simulink model "Gen_net_5"  (R2018b)
settings: Solver=FixedStepAuto  StartTime=0.0  StopTime=100  FixedStep=0.1  RelTol=1e-3
undefined symbols (not defined in the file): g, Jx, Jy, Jz, m, phi_DoS_duration_1, phi_DoS_duration_2, phi_DoS_duration_3, phi_DoS_duration_4, phi_DoS_duration_5, phi_FDI_value_1, phi_FDI_value_2, phi_FDI_value_3, phi_FDI_value_4, phi_FDI_value_5, phi_Replay_delay_1, phi_Replay_delay_2, phi_Replay_delay_3, phi_Replay_delay_4, phi_Replay_delay_5, psi_DoS_duration_1, psi_DoS_duration_2, psi_DoS_duration_3, psi_DoS_duration_4, psi_DoS_duration_5, psi_FDI_value_1, psi_FDI_value_2, psi_FDI_value_3, psi_FDI_value_4, psi_FDI_value_5, psi_Replay_delay_1, psi_Replay_delay_2, psi_Replay_delay_3, psi_Replay_delay_4, psi_Replay_delay_5, T_DoS_duration_1, T_DoS_duration_2, T_DoS_duration_3, T_DoS_duration_4, T_DoS_duration_5, T_FDI_value_1, T_FDI_value_2, T_FDI_value_3, T_FDI_value_4, T_FDI_value_5, T_Replay_delay_1, T_Replay_delay_2, T_Replay_delay_3, T_Replay_delay_4, T_Replay_delay_5, tau_phi_DoS_duration_1, tau_phi_DoS_duration_2, tau_phi_DoS_duration_3, tau_phi_DoS_duration_4, tau_phi_DoS_duration_5, tau_phi_FDI_value_1, tau_phi_FDI_value_2, tau_phi_FDI_value_3, tau_phi_FDI_value_4, tau_phi_FDI_value_5 ... (+95)
libraries: simulink x30
(part 3 of 4)

== system Gen_net_5/quad 2/quadcopter/S(7-9) ==
  phi : Inport
  theta : Inport  Port=2
  q : Inport  Port=3
  P : Inport  Port=4
  r : Inport  Port=5
  Add2 : Sum  Inputs=++-
  Add3 : Sum
  Cos{6..9} (4 alike) : Trigonometry  Operator=cos
  Multiply3 : Product  Inputs=3
  Multiply4 : Product  Inputs=3
  Multiply5 : Product  Inputs=**/
  Multiply6 : Product  Inputs=**/
  Product5 : Product
  Product6 : Product
  Sin6 : Trigonometry
  Sin7 : Trigonometry
  Sin8 : Trigonometry
  Sin9 : Trigonometry  Operator=cos
  Subtract1 : Sum  Inputs=-+
  Tan : Trigonometry  Operator=tan
  Tan1 : Trigonometry  Operator=tan
  Out1 : Outport
  Out2 : Outport  Port=2
  Out3 : Outport  Port=3
  wires:
  Multiply5/1 -> Subtract1/1
  q/1 -> Multiply5/1, Product5/1, Multiply4/3
  phi/1 -> Sin9/1, Sin8/1, Sin7/1, Cos7/1, Cos6/1, Sin6/1
  Multiply4/1 -> Add2/2
  theta/1 -> Cos9/1, Cos8/1, Tan/1, Tan1/1
  Tan/1 -> Multiply4/2
  r/1 -> Multiply6/1, Product6/1, Multiply3/3
  Multiply6/1 -> Subtract1/2
  Sin9/1 -> Multiply6/2
  Sin6/1 -> Multiply4/1
  Sin8/1 -> Multiply5/2
  Tan1/1 -> Multiply3/2
  Product5/1 -> Add3/1
  Cos6/1 -> Multiply3/1
  Product6/1 -> Add3/2
  Sin7/1 -> Product6/2
  Multiply3/1 -> Add2/3
  Cos7/1 -> Product5/2
  Cos8/1 -> Multiply5/3
  Cos9/1 -> Multiply6/3
  Subtract1/1 -> Out3/1
  P/1 -> Add2/1
  Add2/1 -> Out1/1
  Add3/1 -> Out2/1

== system Gen_net_5/quad 3/controller/altitude controller ==
  z_ref : Inport
  z : Inport  Port=2
  Constant : Constant  Value=m*g
  PID Controller : simulink/Continuous/PID Controller  Controller=PID  Form=Parallel  TimeDomain=Continuous-time  SampleTime=-1  IntegratorMethod=Forward Euler  FilterMethod=Forward Euler  ControllerParametersSource=internal  P=0.995151437850186  I=0.128436617904908  D=1.76652121748459  UseFilter=on  N=3.43027649580308  TunerSelectOption=Transfer Function Based (PID Tuner App)  InitialConditionSource=internal  InitialConditionForIntegrator=0  InitialConditionForFilter=0  DifferentiatorICPrevScaledInput=0  ExternalReset=none  TrackingMode=off  Kt=1  LimitOutput=off  UpperSaturationLimit=inf  LowerSaturationLimit=-inf  LinearizeAsGain=on  AntiWindupMode=none  Kb=1  POutMin=[]  POutMax=[]  IOutMin=[]  IOutMax=[]  DOutMin=[]  DOutMax=[]  NOutMin=[]  NOutMax=[]  SumOutMin=[]  SumOutMax=[]  SaturationOutMin=[]  SaturationOutMax=[]  PParamMin=[]  PParamMax=[]  IParamMin=[]  IParamMax=[]  DParamMin=[]  DParamMax=[]  NParamMin=[]  NParamMax=[]  KbParamMin=[]  KbParamMax=[]  KtParamMin=[]  KtParamMax=[]  KbOutMin=[]  KbOutMax=[]  KtOutMin=[]  KtOutMax=[]  IntegratorOutMin=[]  IntegratorOutMax=[]  FilterOutMin=[]  FilterOutMax=[]  SumI1OutMin=[]  SumI1OutMax=[]  SumI2OutMin=[]  SumI2OutMax=[]  SumI3OutMin=[]  SumI3OutMax=[]  SumI4OutMin=[]  SumI4OutMax=[]  SumDOutMin=[]  SumDOutMax=[]  DifferentiatorOutMin=[]  DifferentiatorOutMax=[]  FilterDiffOutCoefMin=[]  FilterDiffOutCoefMax=[]  ReciprocalOutMin=[]  ReciprocalOutMax=[]  SumDenOutMin=[]  SumDenOutMax=[]  SumNumOutMin=[]  SumNumOutMax=[]  DivideOutMin=[]  DivideOutMax=[]  IntegratorContinuousStateAttributes=''  IntegratorStateMustResolveToSignalObject=off  IntegratorRTWStateStorageClass=Auto  FilterContinuousStateAttributes=''  FilterStateMustResolveToSignalObject=off  FilterRTWStateStorageClass=Auto  ParallelPVariant=InternalParameters  IdealPVariant=Disabled  IVariant=InternalParameters  DVariant=InternalParameters  IntegratorVariant=Continuous  SatVariant=Disabled  AWVariant=Passthrough  PCopyVariant=Disabled  TRVariant=Disabled  FdbkBlocksVariant=Forward  IdealPFdbkVariant=Disabled  SatFdbkVariant=Disabled  DerivativeFilterVariant=ContFilter  NVariant=InternalParameters  NCopyVariant=Disabled  FilterICVariant=InternalICsFilter  IntegratorICVariant=InternalICs  ExternalResetVariant=Disabled  TRSumVariant=Passthrough  SumFdbkVariant=Disabled  SumVariant=Sum_PID
  Sum1 : Sum  Inputs=++|
  Sum2 : Sum  Inputs=-+|
  T : Outport
  wires:
  z_ref/1 -> Sum2/2  "z_ref"
  Sum2/1 -> PID Controller/1  "z_err"
  z/1 -> Sum2/1  "z"
  PID Controller/1 -> Sum1/2
  Sum1/1 -> T/1  "z_err"
  Constant/1 -> Sum1/1

== system Gen_net_5/quad 3/controller/attitude controller ==
  phi : Inport
  theta : Inport  Port=2
  phi_ref : Inport  Port=3
  theta_ref : Inport  Port=4
  PID Controller1 : simulink/Continuous/PID Controller  Controller=PID  Form=Parallel  TimeDomain=Continuous-time  SampleTime=-1  IntegratorMethod=Forward Euler  FilterMethod=Forward Euler  ControllerParametersSource=internal  P=0.00283727985172173  I=0.000300746607233676  D=0.00592713753900793  UseFilter=on  N=3.27588862149554  TunerSelectOption=Transfer Function Based (PID Tuner App)  InitialConditionSource=internal  InitialConditionForIntegrator=0  InitialConditionForFilter=0  DifferentiatorICPrevScaledInput=0  ExternalReset=none  TrackingMode=off  Kt=1  LimitOutput=off  UpperSaturationLimit=inf  LowerSaturationLimit=-inf  LinearizeAsGain=on  AntiWindupMode=none  Kb=1  POutMin=[]  POutMax=[]  IOutMin=[]  IOutMax=[]  DOutMin=[]  DOutMax=[]  NOutMin=[]  NOutMax=[]  SumOutMin=[]  SumOutMax=[]  SaturationOutMin=[]  SaturationOutMax=[]  PParamMin=[]  PParamMax=[]  IParamMin=[]  IParamMax=[]  DParamMin=[]  DParamMax=[]  NParamMin=[]  NParamMax=[]  KbParamMin=[]  KbParamMax=[]  KtParamMin=[]  KtParamMax=[]  KbOutMin=[]  KbOutMax=[]  KtOutMin=[]  KtOutMax=[]  IntegratorOutMin=[]  IntegratorOutMax=[]  FilterOutMin=[]  FilterOutMax=[]  SumI1OutMin=[]  SumI1OutMax=[]  SumI2OutMin=[]  SumI2OutMax=[]  SumI3OutMin=[]  SumI3OutMax=[]  SumI4OutMin=[]  SumI4OutMax=[]  SumDOutMin=[]  SumDOutMax=[]  DifferentiatorOutMin=[]  DifferentiatorOutMax=[]  FilterDiffOutCoefMin=[]  FilterDiffOutCoefMax=[]  ReciprocalOutMin=[]  ReciprocalOutMax=[]  SumDenOutMin=[]  SumDenOutMax=[]  SumNumOutMin=[]  SumNumOutMax=[]  DivideOutMin=[]  DivideOutMax=[]  IntegratorContinuousStateAttributes=''  IntegratorStateMustResolveToSignalObject=off  IntegratorRTWStateStorageClass=Auto  FilterContinuousStateAttributes=''  FilterStateMustResolveToSignalObject=off  FilterRTWStateStorageClass=Auto  ParallelPVariant=InternalParameters  IdealPVariant=Disabled  IVariant=InternalParameters  DVariant=InternalParameters  IntegratorVariant=Continuous  SatVariant=Disabled  AWVariant=Passthrough  PCopyVariant=Disabled  TRVariant=Disabled  FdbkBlocksVariant=Forward  IdealPFdbkVariant=Disabled  SatFdbkVariant=Disabled  DerivativeFilterVariant=ContFilter  NVariant=InternalParameters  NCopyVariant=Disabled  FilterICVariant=InternalICsFilter  IntegratorICVariant=InternalICs  ExternalResetVariant=Disabled  TRSumVariant=Passthrough  SumFdbkVariant=Disabled  SumVariant=Sum_PID
  PID Controller2 : simulink/Continuous/PID Controller  Controller=PID  Form=Parallel  TimeDomain=Continuous-time  SampleTime=-1  IntegratorMethod=Forward Euler  FilterMethod=Forward Euler  ControllerParametersSource=internal  P=0.00376352907272366  I=0.000541941810599823  D=0.00599672187002239  UseFilter=on  N=3.43027649580308  TunerSelectOption=Transfer Function Based (PID Tuner App)  InitialConditionSource=internal  InitialConditionForIntegrator=0  InitialConditionForFilter=0  DifferentiatorICPrevScaledInput=0  ExternalReset=none  TrackingMode=off  Kt=1  LimitOutput=off  UpperSaturationLimit=inf  LowerSaturationLimit=-inf  LinearizeAsGain=on  AntiWindupMode=none  Kb=1  POutMin=[]  POutMax=[]  IOutMin=[]  IOutMax=[]  DOutMin=[]  DOutMax=[]  NOutMin=[]  NOutMax=[]  SumOutMin=[]  SumOutMax=[]  SaturationOutMin=[]  SaturationOutMax=[]  PParamMin=[]  PParamMax=[]  IParamMin=[]  IParamMax=[]  DParamMin=[]  DParamMax=[]  NParamMin=[]  NParamMax=[]  KbParamMin=[]  KbParamMax=[]  KtParamMin=[]  KtParamMax=[]  KbOutMin=[]  KbOutMax=[]  KtOutMin=[]  KtOutMax=[]  IntegratorOutMin=[]  IntegratorOutMax=[]  FilterOutMin=[]  FilterOutMax=[]  SumI1OutMin=[]  SumI1OutMax=[]  SumI2OutMin=[]  SumI2OutMax=[]  SumI3OutMin=[]  SumI3OutMax=[]  SumI4OutMin=[]  SumI4OutMax=[]  SumDOutMin=[]  SumDOutMax=[]  DifferentiatorOutMin=[]  DifferentiatorOutMax=[]  FilterDiffOutCoefMin=[]  FilterDiffOutCoefMax=[]  ReciprocalOutMin=[]  ReciprocalOutMax=[]  SumDenOutMin=[]  SumDenOutMax=[]  SumNumOutMin=[]  SumNumOutMax=[]  DivideOutMin=[]  DivideOutMax=[]  IntegratorContinuousStateAttributes=''  IntegratorStateMustResolveToSignalObject=off  IntegratorRTWStateStorageClass=Auto  FilterContinuousStateAttributes=''  FilterStateMustResolveToSignalObject=off  FilterRTWStateStorageClass=Auto  ParallelPVariant=InternalParameters  IdealPVariant=Disabled  IVariant=InternalParameters  DVariant=InternalParameters  IntegratorVariant=Continuous  SatVariant=Disabled  AWVariant=Passthrough  PCopyVariant=Disabled  TRVariant=Disabled  FdbkBlocksVariant=Forward  IdealPFdbkVariant=Disabled  SatFdbkVariant=Disabled  DerivativeFilterVariant=ContFilter  NVariant=InternalParameters  NCopyVariant=Disabled  FilterICVariant=InternalICsFilter  IntegratorICVariant=InternalICs  ExternalResetVariant=Disabled  TRSumVariant=Passthrough  SumFdbkVariant=Disabled  SumVariant=Sum_PID
  Sum1 : Sum  Inputs=-+|
  Sum2 : Sum  Inputs=-+|
  tau_phi : Outport
  tau_theta : Outport  Port=2
  wires:
  phi/1 -> Sum2/1
  theta/1 -> Sum1/1
  phi_ref/1 -> Sum2/2
  theta_ref/1 -> Sum1/2
  Sum1/1 -> PID Controller2/1
  PID Controller2/1 -> tau_theta/1
  Sum2/1 -> PID Controller1/1
  PID Controller1/1 -> tau_phi/1

== system Gen_net_5/quad 3/controller/position controller ==
  x_ref : Inport
  x : Inport  Port=2
  y_ref : Inport  Port=3
  y : Inport  Port=4
  PID Controller : simulink/Continuous/PID Controller  Controller=PID  Form=Parallel  TimeDomain=Continuous-time  SampleTime=-1  IntegratorMethod=Forward Euler  FilterMethod=Forward Euler  ControllerParametersSource=internal  P=-0.0353666022144165  I=-0.000286794158433156  D=-0.0628063352706131  UseFilter=on  N=2.54551622754876  TunerSelectOption=Transfer Function Based (PID Tuner App)  InitialConditionSource=internal  InitialConditionForIntegrator=0  InitialConditionForFilter=0  DifferentiatorICPrevScaledInput=0  ExternalReset=none  TrackingMode=off  Kt=1  LimitOutput=off  UpperSaturationLimit=inf  LowerSaturationLimit=-inf  LinearizeAsGain=on  AntiWindupMode=none  Kb=1  POutMin=[]  POutMax=[]  IOutMin=[]  IOutMax=[]  DOutMin=[]  DOutMax=[]  NOutMin=[]  NOutMax=[]  SumOutMin=[]  SumOutMax=[]  SaturationOutMin=[]  SaturationOutMax=[]  PParamMin=[]  PParamMax=[]  IParamMin=[]  IParamMax=[]  DParamMin=[]  DParamMax=[]  NParamMin=[]  NParamMax=[]  KbParamMin=[]  KbParamMax=[]  KtParamMin=[]  KtParamMax=[]  KbOutMin=[]  KbOutMax=[]  KtOutMin=[]  KtOutMax=[]  IntegratorOutMin=[]  IntegratorOutMax=[]  FilterOutMin=[]  FilterOutMax=[]  SumI1OutMin=[]  SumI1OutMax=[]  SumI2OutMin=[]  SumI2OutMax=[]  SumI3OutMin=[]  SumI3OutMax=[]  SumI4OutMin=[]  SumI4OutMax=[]  SumDOutMin=[]  SumDOutMax=[]  DifferentiatorOutMin=[]  DifferentiatorOutMax=[]  FilterDiffOutCoefMin=[]  FilterDiffOutCoefMax=[]  ReciprocalOutMin=[]  ReciprocalOutMax=[]  SumDenOutMin=[]  SumDenOutMax=[]  SumNumOutMin=[]  SumNumOutMax=[]  DivideOutMin=[]  DivideOutMax=[]  IntegratorContinuousStateAttributes=''  IntegratorStateMustResolveToSignalObject=off  IntegratorRTWStateStorageClass=Auto  FilterContinuousStateAttributes=''  FilterStateMustResolveToSignalObject=off  FilterRTWStateStorageClass=Auto  ParallelPVariant=InternalParameters  IdealPVariant=Disabled  IVariant=InternalParameters  DVariant=InternalParameters  IntegratorVariant=Continuous  SatVariant=Disabled  AWVariant=Passthrough  PCopyVariant=Disabled  TRVariant=Disabled  FdbkBlocksVariant=Forward  IdealPFdbkVariant=Disabled  SatFdbkVariant=Disabled  DerivativeFilterVariant=ContFilter  NVariant=InternalParameters  NCopyVariant=Disabled  FilterICVariant=InternalICsFilter  IntegratorICVariant=InternalICs  ExternalResetVariant=Disabled  TRSumVariant=Passthrough  SumFdbkVariant=Disabled  SumVariant=Sum_PID
  PID Controller1 : simulink/Continuous/PID Controller  Controller=PID  Form=Parallel  TimeDomain=Continuous-time  SampleTime=-1  IntegratorMethod=Forward Euler  FilterMethod=Forward Euler  ControllerParametersSource=internal  P=0.0344011339376346  I=0.00030706355489176  D=0.0770084502146799  UseFilter=on  N=2.81850869669594  TunerSelectOption=Transfer Function Based (PID Tuner App)  InitialConditionSource=internal  InitialConditionForIntegrator=0  InitialConditionForFilter=0  DifferentiatorICPrevScaledInput=0  ExternalReset=none  TrackingMode=off  Kt=1  LimitOutput=off  UpperSaturationLimit=inf  LowerSaturationLimit=-inf  LinearizeAsGain=on  AntiWindupMode=none  Kb=1  POutMin=[]  POutMax=[]  IOutMin=[]  IOutMax=[]  DOutMin=[]  DOutMax=[]  NOutMin=[]  NOutMax=[]  SumOutMin=[]  SumOutMax=[]  SaturationOutMin=[]  SaturationOutMax=[]  PParamMin=[]  PParamMax=[]  IParamMin=[]  IParamMax=[]  DParamMin=[]  DParamMax=[]  NParamMin=[]  NParamMax=[]  KbParamMin=[]  KbParamMax=[]  KtParamMin=[]  KtParamMax=[]  KbOutMin=[]  KbOutMax=[]  KtOutMin=[]  KtOutMax=[]  IntegratorOutMin=[]  IntegratorOutMax=[]  FilterOutMin=[]  FilterOutMax=[]  SumI1OutMin=[]  SumI1OutMax=[]  SumI2OutMin=[]  SumI2OutMax=[]  SumI3OutMin=[]  SumI3OutMax=[]  SumI4OutMin=[]  SumI4OutMax=[]  SumDOutMin=[]  SumDOutMax=[]  DifferentiatorOutMin=[]  DifferentiatorOutMax=[]  FilterDiffOutCoefMin=[]  FilterDiffOutCoefMax=[]  ReciprocalOutMin=[]  ReciprocalOutMax=[]  SumDenOutMin=[]  SumDenOutMax=[]  SumNumOutMin=[]  SumNumOutMax=[]  DivideOutMin=[]  DivideOutMax=[]  IntegratorContinuousStateAttributes=''  IntegratorStateMustResolveToSignalObject=off  IntegratorRTWStateStorageClass=Auto  FilterContinuousStateAttributes=''  FilterStateMustResolveToSignalObject=off  FilterRTWStateStorageClass=Auto  ParallelPVariant=InternalParameters  IdealPVariant=Disabled  IVariant=InternalParameters  DVariant=InternalParameters  IntegratorVariant=Continuous  SatVariant=Disabled  AWVariant=Passthrough  PCopyVariant=Disabled  TRVariant=Disabled  FdbkBlocksVariant=Forward  IdealPFdbkVariant=Disabled  SatFdbkVariant=Disabled  DerivativeFilterVariant=ContFilter  NVariant=InternalParameters  NCopyVariant=Disabled  FilterICVariant=InternalICsFilter  IntegratorICVariant=InternalICs  ExternalResetVariant=Disabled  TRSumVariant=Passthrough  SumFdbkVariant=Disabled  SumVariant=Sum_PID
  Sum1 : Sum  Inputs=-+|
  Sum2 : Sum  Inputs=-+|
  phi_ref : Outport
  theta_ref : Outport  Port=2
  wires:
  x_ref/1 -> Sum2/2
  x/1 -> Sum2/1
  Sum2/1 -> PID Controller/1
  PID Controller/1 -> theta_ref/1
  Sum1/1 -> PID Controller1/1
  y_ref/1 -> Sum1/2
  y/1 -> Sum1/1
  PID Controller1/1 -> phi_ref/1

== system Gen_net_5/quad 3/controller/yaw controller ==
  yaw : Inport
  Constant : Constant  Value=0
  PID Controller3 : simulink/Continuous/PID Controller  Controller=PID  Form=Parallel  TimeDomain=Continuous-time  SampleTime=-1  IntegratorMethod=Forward Euler  FilterMethod=Forward Euler  ControllerParametersSource=internal  P=0.00651371850229212  I=0.000840676044468491  D=0.0115626843326264  UseFilter=on  N=3.43027649580308  TunerSelectOption=Transfer Function Based (PID Tuner App)  InitialConditionSource=internal  InitialConditionForIntegrator=0  InitialConditionForFilter=0  DifferentiatorICPrevScaledInput=0  ExternalReset=none  TrackingMode=off  Kt=1  LimitOutput=off  UpperSaturationLimit=inf  LowerSaturationLimit=-inf  LinearizeAsGain=on  AntiWindupMode=none  Kb=1  POutMin=[]  POutMax=[]  IOutMin=[]  IOutMax=[]  DOutMin=[]  DOutMax=[]  NOutMin=[]  NOutMax=[]  SumOutMin=[]  SumOutMax=[]  SaturationOutMin=[]  SaturationOutMax=[]  PParamMin=[]  PParamMax=[]  IParamMin=[]  IParamMax=[]  DParamMin=[]  DParamMax=[]  NParamMin=[]  NParamMax=[]  KbParamMin=[]  KbParamMax=[]  KtParamMin=[]  KtParamMax=[]  KbOutMin=[]  KbOutMax=[]  KtOutMin=[]  KtOutMax=[]  IntegratorOutMin=[]  IntegratorOutMax=[]  FilterOutMin=[]  FilterOutMax=[]  SumI1OutMin=[]  SumI1OutMax=[]  SumI2OutMin=[]  SumI2OutMax=[]  SumI3OutMin=[]  SumI3OutMax=[]  SumI4OutMin=[]  SumI4OutMax=[]  SumDOutMin=[]  SumDOutMax=[]  DifferentiatorOutMin=[]  DifferentiatorOutMax=[]  FilterDiffOutCoefMin=[]  FilterDiffOutCoefMax=[]  ReciprocalOutMin=[]  ReciprocalOutMax=[]  SumDenOutMin=[]  SumDenOutMax=[]  SumNumOutMin=[]  SumNumOutMax=[]  DivideOutMin=[]  DivideOutMax=[]  IntegratorContinuousStateAttributes=''  IntegratorStateMustResolveToSignalObject=off  IntegratorRTWStateStorageClass=Auto  FilterContinuousStateAttributes=''  FilterStateMustResolveToSignalObject=off  FilterRTWStateStorageClass=Auto  ParallelPVariant=InternalParameters  IdealPVariant=Disabled  IVariant=InternalParameters  DVariant=InternalParameters  IntegratorVariant=Continuous  SatVariant=Disabled  AWVariant=Passthrough  PCopyVariant=Disabled  TRVariant=Disabled  FdbkBlocksVariant=Forward  IdealPFdbkVariant=Disabled  SatFdbkVariant=Disabled  DerivativeFilterVariant=ContFilter  NVariant=InternalParameters  NCopyVariant=Disabled  FilterICVariant=InternalICsFilter  IntegratorICVariant=InternalICs  ExternalResetVariant=Disabled  TRSumVariant=Passthrough  SumFdbkVariant=Disabled  SumVariant=Sum_PID
  Sum2 : Sum  Inputs=-+|
  tau_psi : Outport
  wires:
  yaw/1 -> Sum2/1
  Constant/1 -> Sum2/2
  Sum2/1 -> PID Controller3/1
  PID Controller3/1 -> tau_psi/1

== system Gen_net_5/quad 3/quadcopter/S(10-12) ==
  q : Inport
  P : Inport  Port=2
  r : Inport  Port=3
  In4 : Inport  Port=4
  In5 : Inport  Port=5
  In6 : Inport  Port=6
  Add4 : Sum
  Add5 : Sum
  Add6 : Sum
  Constant4 : Constant  Value=(Jy - Jz) / Jx
  Constant5 : Constant  Value=Jx
  Constant6 : Constant  Value=(Jz - Jx) / Jy
  Constant7 : Constant  Value=Jy
  Constant8 : Constant  Value=(Jx - Jy) / Jz
  Constant9 : Constant  Value=Jz
  Multiply10 : Product  Inputs=*/
  Multiply11 : Product  Inputs=*/
  Multiply12 : Product  Inputs=3
  Multiply7 : Product  Inputs=3
  Multiply8 : Product  Inputs=*/
  Multiply9 : Product  Inputs=3
  Out1 : Outport
  Out2 : Outport  Port=2
  Out3 : Outport  Port=3
  wires:
  r/1 -> Multiply9/3, Multiply7/3
  Constant8/1 -> Multiply12/1
  In5/1 -> Multiply10/1
  Multiply8/1 -> Add4/2
  Multiply7/1 -> Add4/1
  Constant7/1 -> Multiply10/2
  Constant5/1 -> Multiply8/2
  Constant4/1 -> Multiply7/1
  q/1 -> Multiply7/2, Multiply12/3
  Multiply10/1 -> Add5/2
  Multiply9/1 -> Add5/1
  Constant9/1 -> Multiply11/2
  In6/1 -> Multiply11/1
  Constant6/1 -> Multiply9/1
  Multiply12/1 -> Add6/1
  P/1 -> Multiply9/2, Multiply12/2
  In4/1 -> Multiply8/1
  Multiply11/1 -> Add6/2
  Add4/1 -> Out1/1
  Add5/1 -> Out2/1
  Add6/1 -> Out3/1

== system Gen_net_5/quad 3/quadcopter/S(4-6) ==
  In1 : Inport
  phi : Inport  Port=2
  theta : Inport  Port=3
  psi : Inport  Port=4
  Add : Sum  Inputs=--
  Add1 : Sum  Inputs=+-
  Constant1 : Constant  Value=0.0
  Constant3 : Constant  Value=g
  Cos{,1..5} (6 alike) : Trigonometry  Operator=cos
  Multiply : Product
  Multiply1 : Product
  Multiply2 : Product
  Product : Product  Inputs=3
  Product1 : Product
  Product2 : Product
  Product3 : Product  Inputs=3
  Product4 : Product
  Sin{,1..5} (6 alike) : Trigonometry
  Subtract : Sum  Inputs=+-
  Sum3 : Sum  Inputs=++|
  Out1 : Outport
  Out2 : Outport  Port=2
  Out3 : Outport  Port=3
  wires:
  phi/1 -> Cos4/1, Cos3/1, Cos1/1, Sin2/1, Sin3/1
  theta/1 -> Sin/1, Sin5/1, Cos5/1
  Sum3/1 -> Out1/1
  Constant1/1 -> Sum3/1
  Product1/1 -> Add/2
  Sin3/1 -> Product2/2
  Cos/1 -> Product/1
  Cos1/1 -> Product/3
  Multiply/1 -> Sum3/2
  Sin/1 -> Product/2
  Cos5/1 -> Product4/2
  psi/1 -> Cos/1, Sin1/1, Cos2/1, Sin4/1
  Cos3/1 -> Product3/3
  Product2/1 -> Add1/1
  Add1/1 -> Multiply1/2
  Sin1/1 -> Product1/1
  Sin4/1 -> Product3/1
  Sin5/1 -> Product3/2
  Cos4/1 -> Product4/1
  Cos2/1 -> Product2/1
  Subtract/1 -> Out3/1
  Sin2/1 -> Product1/2
  Constant3/1 -> Subtract/2
  Product4/1 -> Multiply2/2
  In1/1 -> Multiply2/1, Multiply1/1, Multiply/1
  Add/1 -> Multiply/2
  Product3/1 -> Add1/2
  Multiply2/1 -> Subtract/1
  Product/1 -> Add/1
  Multiply1/1 -> Out2/1

== system Gen_net_5/quad 3/quadcopter/S(7-9) ==
  phi : Inport
  theta : Inport  Port=2
  q : Inport  Port=3
  P : Inport  Port=4
  r : Inport  Port=5
  Add2 : Sum  Inputs=++-
  Add3 : Sum
  Cos{6..9} (4 alike) : Trigonometry  Operator=cos
  Multiply3 : Product  Inputs=3
  Multiply4 : Product  Inputs=3
  Multiply5 : Product  Inputs=**/
  Multiply6 : Product  Inputs=**/
  Product5 : Product
  Product6 : Product
  Sin6 : Trigonometry
  Sin7 : Trigonometry
  Sin8 : Trigonometry
  Sin9 : Trigonometry  Operator=cos
  Subtract1 : Sum  Inputs=-+
  Tan : Trigonometry  Operator=tan
  Tan1 : Trigonometry  Operator=tan
  Out1 : Outport
  Out2 : Outport  Port=2
  Out3 : Outport  Port=3
  wires:
  Multiply5/1 -> Subtract1/1
  q/1 -> Multiply5/1, Product5/1, Multiply4/3
  phi/1 -> Sin9/1, Sin8/1, Sin7/1, Cos7/1, Cos6/1, Sin6/1
  Multiply4/1 -> Add2/2
  theta/1 -> Cos9/1, Cos8/1, Tan/1, Tan1/1
  Tan/1 -> Multiply4/2
  r/1 -> Multiply6/1, Product6/1, Multiply3/3
  Multiply6/1 -> Subtract1/2
  Sin9/1 -> Multiply6/2
  Sin6/1 -> Multiply4/1
  Sin8/1 -> Multiply5/2
  Tan1/1 -> Multiply3/2
  Product5/1 -> Add3/1
  Cos6/1 -> Multiply3/1
  Product6/1 -> Add3/2
  Sin7/1 -> Product6/2
  Multiply3/1 -> Add2/3
  Cos7/1 -> Product5/2
  Cos8/1 -> Multiply5/3
  Cos9/1 -> Multiply6/3
  Subtract1/1 -> Out3/1
  P/1 -> Add2/1
  Add2/1 -> Out1/1
  Add3/1 -> Out2/1

== system Gen_net_5/quad 4/controller/altitude controller ==
  z_ref : Inport
  z : Inport  Port=2
  Constant : Constant  Value=m*g
  PID Controller : simulink/Continuous/PID Controller  Controller=PID  Form=Parallel  TimeDomain=Continuous-time  SampleTime=-1  IntegratorMethod=Forward Euler  FilterMethod=Forward Euler  ControllerParametersSource=internal  P=0.995151437850186  I=0.128436617904908  D=1.76652121748459  UseFilter=on  N=3.43027649580308  TunerSelectOption=Transfer Function Based (PID Tuner App)  InitialConditionSource=internal  InitialConditionForIntegrator=0  InitialConditionForFilter=0  DifferentiatorICPrevScaledInput=0  ExternalReset=none  TrackingMode=off  Kt=1  LimitOutput=off  UpperSaturationLimit=inf  LowerSaturationLimit=-inf  LinearizeAsGain=on  AntiWindupMode=none  Kb=1  POutMin=[]  POutMax=[]  IOutMin=[]  IOutMax=[]  DOutMin=[]  DOutMax=[]  NOutMin=[]  NOutMax=[]  SumOutMin=[]  SumOutMax=[]  SaturationOutMin=[]  SaturationOutMax=[]  PParamMin=[]  PParamMax=[]  IParamMin=[]  IParamMax=[]  DParamMin=[]  DParamMax=[]  NParamMin=[]  NParamMax=[]  KbParamMin=[]  KbParamMax=[]  KtParamMin=[]  KtParamMax=[]  KbOutMin=[]  KbOutMax=[]  KtOutMin=[]  KtOutMax=[]  IntegratorOutMin=[]  IntegratorOutMax=[]  FilterOutMin=[]  FilterOutMax=[]  SumI1OutMin=[]  SumI1OutMax=[]  SumI2OutMin=[]  SumI2OutMax=[]  SumI3OutMin=[]  SumI3OutMax=[]  SumI4OutMin=[]  SumI4OutMax=[]  SumDOutMin=[]  SumDOutMax=[]  DifferentiatorOutMin=[]  DifferentiatorOutMax=[]  FilterDiffOutCoefMin=[]  FilterDiffOutCoefMax=[]  ReciprocalOutMin=[]  ReciprocalOutMax=[]  SumDenOutMin=[]  SumDenOutMax=[]  SumNumOutMin=[]  SumNumOutMax=[]  DivideOutMin=[]  DivideOutMax=[]  IntegratorContinuousStateAttributes=''  IntegratorStateMustResolveToSignalObject=off  IntegratorRTWStateStorageClass=Auto  FilterContinuousStateAttributes=''  FilterStateMustResolveToSignalObject=off  FilterRTWStateStorageClass=Auto  ParallelPVariant=InternalParameters  IdealPVariant=Disabled  IVariant=InternalParameters  DVariant=InternalParameters  IntegratorVariant=Continuous  SatVariant=Disabled  AWVariant=Passthrough  PCopyVariant=Disabled  TRVariant=Disabled  FdbkBlocksVariant=Forward  IdealPFdbkVariant=Disabled  SatFdbkVariant=Disabled  DerivativeFilterVariant=ContFilter  NVariant=InternalParameters  NCopyVariant=Disabled  FilterICVariant=InternalICsFilter  IntegratorICVariant=InternalICs  ExternalResetVariant=Disabled  TRSumVariant=Passthrough  SumFdbkVariant=Disabled  SumVariant=Sum_PID
  Sum1 : Sum  Inputs=++|
  Sum2 : Sum  Inputs=-+|
  T : Outport
  wires:
  z_ref/1 -> Sum2/2  "z_ref"
  Sum2/1 -> PID Controller/1  "z_err"
  z/1 -> Sum2/1  "z"
  PID Controller/1 -> Sum1/2
  Sum1/1 -> T/1  "z_err"
  Constant/1 -> Sum1/1

== system Gen_net_5/quad 4/controller/attitude controller ==
  phi : Inport
  theta : Inport  Port=2
  phi_ref : Inport  Port=3
  theta_ref : Inport  Port=4
  PID Controller1 : simulink/Continuous/PID Controller  Controller=PID  Form=Parallel  TimeDomain=Continuous-time  SampleTime=-1  IntegratorMethod=Forward Euler  FilterMethod=Forward Euler  ControllerParametersSource=internal  P=0.00283727985172173  I=0.000300746607233676  D=0.00592713753900793  UseFilter=on  N=3.27588862149554  TunerSelectOption=Transfer Function Based (PID Tuner App)  InitialConditionSource=internal  InitialConditionForIntegrator=0  InitialConditionForFilter=0  DifferentiatorICPrevScaledInput=0  ExternalReset=none  TrackingMode=off  Kt=1  LimitOutput=off  UpperSaturationLimit=inf  LowerSaturationLimit=-inf  LinearizeAsGain=on  AntiWindupMode=none  Kb=1  POutMin=[]  POutMax=[]  IOutMin=[]  IOutMax=[]  DOutMin=[]  DOutMax=[]  NOutMin=[]  NOutMax=[]  SumOutMin=[]  SumOutMax=[]  SaturationOutMin=[]  SaturationOutMax=[]  PParamMin=[]  PParamMax=[]  IParamMin=[]  IParamMax=[]  DParamMin=[]  DParamMax=[]  NParamMin=[]  NParamMax=[]  KbParamMin=[]  KbParamMax=[]  KtParamMin=[]  KtParamMax=[]  KbOutMin=[]  KbOutMax=[]  KtOutMin=[]  KtOutMax=[]  IntegratorOutMin=[]  IntegratorOutMax=[]  FilterOutMin=[]  FilterOutMax=[]  SumI1OutMin=[]  SumI1OutMax=[]  SumI2OutMin=[]  SumI2OutMax=[]  SumI3OutMin=[]  SumI3OutMax=[]  SumI4OutMin=[]  SumI4OutMax=[]  SumDOutMin=[]  SumDOutMax=[]  DifferentiatorOutMin=[]  DifferentiatorOutMax=[]  FilterDiffOutCoefMin=[]  FilterDiffOutCoefMax=[]  ReciprocalOutMin=[]  ReciprocalOutMax=[]  SumDenOutMin=[]  SumDenOutMax=[]  SumNumOutMin=[]  SumNumOutMax=[]  DivideOutMin=[]  DivideOutMax=[]  IntegratorContinuousStateAttributes=''  IntegratorStateMustResolveToSignalObject=off  IntegratorRTWStateStorageClass=Auto  FilterContinuousStateAttributes=''  FilterStateMustResolveToSignalObject=off  FilterRTWStateStorageClass=Auto  ParallelPVariant=InternalParameters  IdealPVariant=Disabled  IVariant=InternalParameters  DVariant=InternalParameters  IntegratorVariant=Continuous  SatVariant=Disabled  AWVariant=Passthrough  PCopyVariant=Disabled  TRVariant=Disabled  FdbkBlocksVariant=Forward  IdealPFdbkVariant=Disabled  SatFdbkVariant=Disabled  DerivativeFilterVariant=ContFilter  NVariant=InternalParameters  NCopyVariant=Disabled  FilterICVariant=InternalICsFilter  IntegratorICVariant=InternalICs  ExternalResetVariant=Disabled  TRSumVariant=Passthrough  SumFdbkVariant=Disabled  SumVariant=Sum_PID
  PID Controller2 : simulink/Continuous/PID Controller  Controller=PID  Form=Parallel  TimeDomain=Continuous-time  SampleTime=-1  IntegratorMethod=Forward Euler  FilterMethod=Forward Euler  ControllerParametersSource=internal  P=0.00376352907272366  I=0.000541941810599823  D=0.00599672187002239  UseFilter=on  N=3.43027649580308  TunerSelectOption=Transfer Function Based (PID Tuner App)  InitialConditionSource=internal  InitialConditionForIntegrator=0  InitialConditionForFilter=0  DifferentiatorICPrevScaledInput=0  ExternalReset=none  TrackingMode=off  Kt=1  LimitOutput=off  UpperSaturationLimit=inf  LowerSaturationLimit=-inf  LinearizeAsGain=on  AntiWindupMode=none  Kb=1  POutMin=[]  POutMax=[]  IOutMin=[]  IOutMax=[]  DOutMin=[]  DOutMax=[]  NOutMin=[]  NOutMax=[]  SumOutMin=[]  SumOutMax=[]  SaturationOutMin=[]  SaturationOutMax=[]  PParamMin=[]  PParamMax=[]  IParamMin=[]  IParamMax=[]  DParamMin=[]  DParamMax=[]  NParamMin=[]  NParamMax=[]  KbParamMin=[]  KbParamMax=[]  KtParamMin=[]  KtParamMax=[]  KbOutMin=[]  KbOutMax=[]  KtOutMin=[]  KtOutMax=[]  IntegratorOutMin=[]  IntegratorOutMax=[]  FilterOutMin=[]  FilterOutMax=[]  SumI1OutMin=[]  SumI1OutMax=[]  SumI2OutMin=[]  SumI2OutMax=[]  SumI3OutMin=[]  SumI3OutMax=[]  SumI4OutMin=[]  SumI4OutMax=[]  SumDOutMin=[]  SumDOutMax=[]  DifferentiatorOutMin=[]  DifferentiatorOutMax=[]  FilterDiffOutCoefMin=[]  FilterDiffOutCoefMax=[]  ReciprocalOutMin=[]  ReciprocalOutMax=[]  SumDenOutMin=[]  SumDenOutMax=[]  SumNumOutMin=[]  SumNumOutMax=[]  DivideOutMin=[]  DivideOutMax=[]  IntegratorContinuousStateAttributes=''  IntegratorStateMustResolveToSignalObject=off  IntegratorRTWStateStorageClass=Auto  FilterContinuousStateAttributes=''  FilterStateMustResolveToSignalObject=off  FilterRTWStateStorageClass=Auto  ParallelPVariant=InternalParameters  IdealPVariant=Disabled  IVariant=InternalParameters  DVariant=InternalParameters  IntegratorVariant=Continuous  SatVariant=Disabled  AWVariant=Passthrough  PCopyVariant=Disabled  TRVariant=Disabled  FdbkBlocksVariant=Forward  IdealPFdbkVariant=Disabled  SatFdbkVariant=Disabled  DerivativeFilterVariant=ContFilter  NVariant=InternalParameters  NCopyVariant=Disabled  FilterICVariant=InternalICsFilter  IntegratorICVariant=InternalICs  ExternalResetVariant=Disabled  TRSumVariant=Passthrough  SumFdbkVariant=Disabled  SumVariant=Sum_PID
  Sum1 : Sum  Inputs=-+|
  Sum2 : Sum  Inputs=-+|
  tau_phi : Outport
  tau_theta : Outport  Port=2
  wires:
  phi/1 -> Sum2/1
  theta/1 -> Sum1/1
  phi_ref/1 -> Sum2/2
  theta_ref/1 -> Sum1/2
  Sum1/1 -> PID Controller2/1
  PID Controller2/1 -> tau_theta/1
  Sum2/1 -> PID Controller1/1
  PID Controller1/1 -> tau_phi/1

== system Gen_net_5/quad 4/controller/position controller ==
  x_ref : Inport
  x : Inport  Port=2
  y_ref : Inport  Port=3
  y : Inport  Port=4
  PID Controller : simulink/Continuous/PID Controller  Controller=PID  Form=Parallel  TimeDomain=Continuous-time  SampleTime=-1  IntegratorMethod=Forward Euler  FilterMethod=Forward Euler  ControllerParametersSource=internal  P=-0.0353666022144165  I=-0.000286794158433156  D=-0.0628063352706131  UseFilter=on  N=2.54551622754876  TunerSelectOption=Transfer Function Based (PID Tuner App)  InitialConditionSource=internal  InitialConditionForIntegrator=0  InitialConditionForFilter=0  DifferentiatorICPrevScaledInput=0  ExternalReset=none  TrackingMode=off  Kt=1  LimitOutput=off  UpperSaturationLimit=inf  LowerSaturationLimit=-inf  LinearizeAsGain=on  AntiWindupMode=none  Kb=1  POutMin=[]  POutMax=[]  IOutMin=[]  IOutMax=[]  DOutMin=[]  DOutMax=[]  NOutMin=[]  NOutMax=[]  SumOutMin=[]  SumOutMax=[]  SaturationOutMin=[]  SaturationOutMax=[]  PParamMin=[]  PParamMax=[]  IParamMin=[]  IParamMax=[]  DParamMin=[]  DParamMax=[]  NParamMin=[]  NParamMax=[]  KbParamMin=[]  KbParamMax=[]  KtParamMin=[]  KtParamMax=[]  KbOutMin=[]  KbOutMax=[]  KtOutMin=[]  KtOutMax=[]  IntegratorOutMin=[]  IntegratorOutMax=[]  FilterOutMin=[]  FilterOutMax=[]  SumI1OutMin=[]  SumI1OutMax=[]  SumI2OutMin=[]  SumI2OutMax=[]  SumI3OutMin=[]  SumI3OutMax=[]  SumI4OutMin=[]  SumI4OutMax=[]  SumDOutMin=[]  SumDOutMax=[]  DifferentiatorOutMin=[]  DifferentiatorOutMax=[]  FilterDiffOutCoefMin=[]  FilterDiffOutCoefMax=[]  ReciprocalOutMin=[]  ReciprocalOutMax=[]  SumDenOutMin=[]  SumDenOutMax=[]  SumNumOutMin=[]  SumNumOutMax=[]  DivideOutMin=[]  DivideOutMax=[]  IntegratorContinuousStateAttributes=''  IntegratorStateMustResolveToSignalObject=off  IntegratorRTWStateStorageClass=Auto  FilterContinuousStateAttributes=''  FilterStateMustResolveToSignalObject=off  FilterRTWStateStorageClass=Auto  ParallelPVariant=InternalParameters  IdealPVariant=Disabled  IVariant=InternalParameters  DVariant=InternalParameters  IntegratorVariant=Continuous  SatVariant=Disabled  AWVariant=Passthrough  PCopyVariant=Disabled  TRVariant=Disabled  FdbkBlocksVariant=Forward  IdealPFdbkVariant=Disabled  SatFdbkVariant=Disabled  DerivativeFilterVariant=ContFilter  NVariant=InternalParameters  NCopyVariant=Disabled  FilterICVariant=InternalICsFilter  IntegratorICVariant=InternalICs  ExternalResetVariant=Disabled  TRSumVariant=Passthrough  SumFdbkVariant=Disabled  SumVariant=Sum_PID
  PID Controller1 : simulink/Continuous/PID Controller  Controller=PID  Form=Parallel  TimeDomain=Continuous-time  SampleTime=-1  IntegratorMethod=Forward Euler  FilterMethod=Forward Euler  ControllerParametersSource=internal  P=0.0344011339376346  I=0.00030706355489176  D=0.0770084502146799  UseFilter=on  N=2.81850869669594  TunerSelectOption=Transfer Function Based (PID Tuner App)  InitialConditionSource=internal  InitialConditionForIntegrator=0  InitialConditionForFilter=0  DifferentiatorICPrevScaledInput=0  ExternalReset=none  TrackingMode=off  Kt=1  LimitOutput=off  UpperSaturationLimit=inf  LowerSaturationLimit=-inf  LinearizeAsGain=on  AntiWindupMode=none  Kb=1  POutMin=[]  POutMax=[]  IOutMin=[]  IOutMax=[]  DOutMin=[]  DOutMax=[]  NOutMin=[]  NOutMax=[]  SumOutMin=[]  SumOutMax=[]  SaturationOutMin=[]  SaturationOutMax=[]  PParamMin=[]  PParamMax=[]  IParamMin=[]  IParamMax=[]  DParamMin=[]  DParamMax=[]  NParamMin=[]  NParamMax=[]  KbParamMin=[]  KbParamMax=[]  KtParamMin=[]  KtParamMax=[]  KbOutMin=[]  KbOutMax=[]  KtOutMin=[]  KtOutMax=[]  IntegratorOutMin=[]  IntegratorOutMax=[]  FilterOutMin=[]  FilterOutMax=[]  SumI1OutMin=[]  SumI1OutMax=[]  SumI2OutMin=[]  SumI2OutMax=[]  SumI3OutMin=[]  SumI3OutMax=[]  SumI4OutMin=[]  SumI4OutMax=[]  SumDOutMin=[]  SumDOutMax=[]  DifferentiatorOutMin=[]  DifferentiatorOutMax=[]  FilterDiffOutCoefMin=[]  FilterDiffOutCoefMax=[]  ReciprocalOutMin=[]  ReciprocalOutMax=[]  SumDenOutMin=[]  SumDenOutMax=[]  SumNumOutMin=[]  SumNumOutMax=[]  DivideOutMin=[]  DivideOutMax=[]  IntegratorContinuousStateAttributes=''  IntegratorStateMustResolveToSignalObject=off  IntegratorRTWStateStorageClass=Auto  FilterContinuousStateAttributes=''  FilterStateMustResolveToSignalObject=off  FilterRTWStateStorageClass=Auto  ParallelPVariant=InternalParameters  IdealPVariant=Disabled  IVariant=InternalParameters  DVariant=InternalParameters  IntegratorVariant=Continuous  SatVariant=Disabled  AWVariant=Passthrough  PCopyVariant=Disabled  TRVariant=Disabled  FdbkBlocksVariant=Forward  IdealPFdbkVariant=Disabled  SatFdbkVariant=Disabled  DerivativeFilterVariant=ContFilter  NVariant=InternalParameters  NCopyVariant=Disabled  FilterICVariant=InternalICsFilter  IntegratorICVariant=InternalICs  ExternalResetVariant=Disabled  TRSumVariant=Passthrough  SumFdbkVariant=Disabled  SumVariant=Sum_PID
  Sum1 : Sum  Inputs=-+|
  Sum2 : Sum  Inputs=-+|
  phi_ref : Outport
  theta_ref : Outport  Port=2
  wires:
  x_ref/1 -> Sum2/2
  x/1 -> Sum2/1
  Sum2/1 -> PID Controller/1
  PID Controller/1 -> theta_ref/1
  Sum1/1 -> PID Controller1/1
  y_ref/1 -> Sum1/2
  y/1 -> Sum1/1
  PID Controller1/1 -> phi_ref/1

== system Gen_net_5/quad 4/controller/yaw controller ==
  yaw : Inport
  Constant : Constant  Value=0
  PID Controller3 : simulink/Continuous/PID Controller  Controller=PID  Form=Parallel  TimeDomain=Continuous-time  SampleTime=-1  IntegratorMethod=Forward Euler  FilterMethod=Forward Euler  ControllerParametersSource=internal  P=0.00651371850229212  I=0.000840676044468491  D=0.0115626843326264  UseFilter=on  N=3.43027649580308  TunerSelectOption=Transfer Function Based (PID Tuner App)  InitialConditionSource=internal  InitialConditionForIntegrator=0  InitialConditionForFilter=0  DifferentiatorICPrevScaledInput=0  ExternalReset=none  TrackingMode=off  Kt=1  LimitOutput=off  UpperSaturationLimit=inf  LowerSaturationLimit=-inf  LinearizeAsGain=on  AntiWindupMode=none  Kb=1  POutMin=[]  POutMax=[]  IOutMin=[]  IOutMax=[]  DOutMin=[]  DOutMax=[]  NOutMin=[]  NOutMax=[]  SumOutMin=[]  SumOutMax=[]  SaturationOutMin=[]  SaturationOutMax=[]  PParamMin=[]  PParamMax=[]  IParamMin=[]  IParamMax=[]  DParamMin=[]  DParamMax=[]  NParamMin=[]  NParamMax=[]  KbParamMin=[]  KbParamMax=[]  KtParamMin=[]  KtParamMax=[]  KbOutMin=[]  KbOutMax=[]  KtOutMin=[]  KtOutMax=[]  IntegratorOutMin=[]  IntegratorOutMax=[]  FilterOutMin=[]  FilterOutMax=[]  SumI1OutMin=[]  SumI1OutMax=[]  SumI2OutMin=[]  SumI2OutMax=[]  SumI3OutMin=[]  SumI3OutMax=[]  SumI4OutMin=[]  SumI4OutMax=[]  SumDOutMin=[]  SumDOutMax=[]  DifferentiatorOutMin=[]  DifferentiatorOutMax=[]  FilterDiffOutCoefMin=[]  FilterDiffOutCoefMax=[]  ReciprocalOutMin=[]  ReciprocalOutMax=[]  SumDenOutMin=[]  SumDenOutMax=[]  SumNumOutMin=[]  SumNumOutMax=[]  DivideOutMin=[]  DivideOutMax=[]  IntegratorContinuousStateAttributes=''  IntegratorStateMustResolveToSignalObject=off  IntegratorRTWStateStorageClass=Auto  FilterContinuousStateAttributes=''  FilterStateMustResolveToSignalObject=off  FilterRTWStateStorageClass=Auto  ParallelPVariant=InternalParameters  IdealPVariant=Disabled  IVariant=InternalParameters  DVariant=InternalParameters  IntegratorVariant=Continuous  SatVariant=Disabled  AWVariant=Passthrough  PCopyVariant=Disabled  TRVariant=Disabled  FdbkBlocksVariant=Forward  IdealPFdbkVariant=Disabled  SatFdbkVariant=Disabled  DerivativeFilterVariant=ContFilter  NVariant=InternalParameters  NCopyVariant=Disabled  FilterICVariant=InternalICsFilter  IntegratorICVariant=InternalICs  ExternalResetVariant=Disabled  TRSumVariant=Passthrough  SumFdbkVariant=Disabled  SumVariant=Sum_PID
  Sum2 : Sum  Inputs=-+|
  tau_psi : Outport
  wires:
  yaw/1 -> Sum2/1
  Constant/1 -> Sum2/2
  Sum2/1 -> PID Controller3/1
  PID Controller3/1 -> tau_psi/1

== system Gen_net_5/quad 4/quadcopter/S(10-12) ==
  q : Inport
  P : Inport  Port=2
  r : Inport  Port=3
  In4 : Inport  Port=4
  In5 : Inport  Port=5
  In6 : Inport  Port=6
  Add4 : Sum
  Add5 : Sum
  Add6 : Sum
  Constant4 : Constant  Value=(Jy - Jz) / Jx
  Constant5 : Constant  Value=Jx
  Constant6 : Constant  Value=(Jz - Jx) / Jy
  Constant7 : Constant  Value=Jy
  Constant8 : Constant  Value=(Jx - Jy) / Jz
  Constant9 : Constant  Value=Jz
  Multiply10 : Product  Inputs=*/
  Multiply11 : Product  Inputs=*/
  Multiply12 : Product  Inputs=3
  Multiply7 : Product  Inputs=3
  Multiply8 : Product  Inputs=*/
  Multiply9 : Product  Inputs=3
  Out1 : Outport
  Out2 : Outport  Port=2
  Out3 : Outport  Port=3
  wires:
  r/1 -> Multiply9/3, Multiply7/3
  Constant8/1 -> Multiply12/1
  In5/1 -> Multiply10/1
  Multiply8/1 -> Add4/2
  Multiply7/1 -> Add4/1
  Constant7/1 -> Multiply10/2
  Constant5/1 -> Multiply8/2
  Constant4/1 -> Multiply7/1
  q/1 -> Multiply7/2, Multiply12/3
  Multiply10/1 -> Add5/2
  Multiply9/1 -> Add5/1
  Constant9/1 -> Multiply11/2
  In6/1 -> Multiply11/1
  Constant6/1 -> Multiply9/1
  Multiply12/1 -> Add6/1
  P/1 -> Multiply9/2, Multiply12/2
  In4/1 -> Multiply8/1
  Multiply11/1 -> Add6/2
  Add4/1 -> Out1/1
  Add5/1 -> Out2/1
  Add6/1 -> Out3/1

== system Gen_net_5/quad 4/quadcopter/S(4-6) ==
  In1 : Inport
  phi : Inport  Port=2
  theta : Inport  Port=3
  psi : Inport  Port=4
  Add : Sum  Inputs=--
  Add1 : Sum  Inputs=+-
  Constant1 : Constant  Value=0.0
  Constant3 : Constant  Value=g
  Cos{,1..5} (6 alike) : Trigonometry  Operator=cos
  Multiply : Product
  Multiply1 : Product
  Multiply2 : Product
  Product : Product  Inputs=3
  Product1 : Product
  Product2 : Product
  Product3 : Product  Inputs=3
  Product4 : Product
  Sin{,1..5} (6 alike) : Trigonometry
  Subtract : Sum  Inputs=+-
  Sum3 : Sum  Inputs=++|
  Out1 : Outport
  Out2 : Outport  Port=2
  Out3 : Outport  Port=3
  wires:
  phi/1 -> Cos4/1, Cos3/1, Cos1/1, Sin2/1, Sin3/1
  theta/1 -> Sin/1, Sin5/1, Cos5/1
  Sum3/1 -> Out1/1
  Constant1/1 -> Sum3/1
  Product1/1 -> Add/2
  Sin3/1 -> Product2/2
  Cos/1 -> Product/1
  Cos1/1 -> Product/3
  Multiply/1 -> Sum3/2
  Sin/1 -> Product/2
  Cos5/1 -> Product4/2
  psi/1 -> Cos/1, Sin1/1, Cos2/1, Sin4/1
  Cos3/1 -> Product3/3
  Product2/1 -> Add1/1
  Add1/1 -> Multiply1/2
  Sin1/1 -> Product1/1
  Sin4/1 -> Product3/1
  Sin5/1 -> Product3/2
  Cos4/1 -> Product4/1
  Cos2/1 -> Product2/1
  Subtract/1 -> Out3/1
  Sin2/1 -> Product1/2
  Constant3/1 -> Subtract/2
  Product4/1 -> Multiply2/2
  In1/1 -> Multiply2/1, Multiply1/1, Multiply/1
  Add/1 -> Multiply/2
  Product3/1 -> Add1/2
  Multiply2/1 -> Subtract/1
  Product/1 -> Add/1
  Multiply1/1 -> Out2/1

== system Gen_net_5/quad 4/quadcopter/S(7-9) ==
  phi : Inport
  theta : Inport  Port=2
  q : Inport  Port=3
  P : Inport  Port=4
  r : Inport  Port=5
  Add2 : Sum  Inputs=++-
  Add3 : Sum
  Cos{6..9} (4 alike) : Trigonometry  Operator=cos
  Multiply3 : Product  Inputs=3
  Multiply4 : Product  Inputs=3
  Multiply5 : Product  Inputs=**/
  Multiply6 : Product  Inputs=**/
  Product5 : Product
  Product6 : Product
  Sin6 : Trigonometry
  Sin7 : Trigonometry
  Sin8 : Trigonometry
  Sin9 : Trigonometry  Operator=cos
  Subtract1 : Sum  Inputs=-+
  Tan : Trigonometry  Operator=tan
  Tan1 : Trigonometry  Operator=tan
  Out1 : Outport
  Out2 : Outport  Port=2
  Out3 : Outport  Port=3
  wires:
  Multiply5/1 -> Subtract1/1
  q/1 -> Multiply5/1, Product5/1, Multiply4/3
  phi/1 -> Sin9/1, Sin8/1, Sin7/1, Cos7/1, Cos6/1, Sin6/1
  Multiply4/1 -> Add2/2
  theta/1 -> Cos9/1, Cos8/1, Tan/1, Tan1/1
  Tan/1 -> Multiply4/2
  r/1 -> Multiply6/1, Product6/1, Multiply3/3
  Multiply6/1 -> Subtract1/2
  Sin9/1 -> Multiply6/2
  Sin6/1 -> Multiply4/1
  Sin8/1 -> Multiply5/2
  Tan1/1 -> Multiply3/2
  Product5/1 -> Add3/1
  Cos6/1 -> Multiply3/1
  Product6/1 -> Add3/2
  Sin7/1 -> Product6/2
  Multiply3/1 -> Add2/3
  Cos7/1 -> Product5/2
  Cos8/1 -> Multiply5/3
  Cos9/1 -> Multiply6/3
  Subtract1/1 -> Out3/1
  P/1 -> Add2/1
  Add2/1 -> Out1/1
  Add3/1 -> Out2/1

== system Gen_net_5/quad 5/controller/altitude controller ==
  z_ref : Inport
  z : Inport  Port=2
  Constant : Constant  Value=m*g
  PID Controller : simulink/Continuous/PID Controller  Controller=PID  Form=Parallel  TimeDomain=Continuous-time  SampleTime=-1  IntegratorMethod=Forward Euler  FilterMethod=Forward Euler  ControllerParametersSource=internal  P=0.995151437850186  I=0.128436617904908  D=1.76652121748459  UseFilter=on  N=3.43027649580308  TunerSelectOption=Transfer Function Based (PID Tuner App)  InitialConditionSource=internal  InitialConditionForIntegrator=0  InitialConditionForFilter=0  DifferentiatorICPrevScaledInput=0  ExternalReset=none  TrackingMode=off  Kt=1  LimitOutput=off  UpperSaturationLimit=inf  LowerSaturationLimit=-inf  LinearizeAsGain=on  AntiWindupMode=none  Kb=1  POutMin=[]  POutMax=[]  IOutMin=[]  IOutMax=[]  DOutMin=[]  DOutMax=[]  NOutMin=[]  NOutMax=[]  SumOutMin=[]  SumOutMax=[]  SaturationOutMin=[]  SaturationOutMax=[]  PParamMin=[]  PParamMax=[]  IParamMin=[]  IParamMax=[]  DParamMin=[]  DParamMax=[]  NParamMin=[]  NParamMax=[]  KbParamMin=[]  KbParamMax=[]  KtParamMin=[]  KtParamMax=[]  KbOutMin=[]  KbOutMax=[]  KtOutMin=[]  KtOutMax=[]  IntegratorOutMin=[]  IntegratorOutMax=[]  FilterOutMin=[]  FilterOutMax=[]  SumI1OutMin=[]  SumI1OutMax=[]  SumI2OutMin=[]  SumI2OutMax=[]  SumI3OutMin=[]  SumI3OutMax=[]  SumI4OutMin=[]  SumI4OutMax=[]  SumDOutMin=[]  SumDOutMax=[]  DifferentiatorOutMin=[]  DifferentiatorOutMax=[]  FilterDiffOutCoefMin=[]  FilterDiffOutCoefMax=[]  ReciprocalOutMin=[]  ReciprocalOutMax=[]  SumDenOutMin=[]  SumDenOutMax=[]  SumNumOutMin=[]  SumNumOutMax=[]  DivideOutMin=[]  DivideOutMax=[]  IntegratorContinuousStateAttributes=''  IntegratorStateMustResolveToSignalObject=off  IntegratorRTWStateStorageClass=Auto  FilterContinuousStateAttributes=''  FilterStateMustResolveToSignalObject=off  FilterRTWStateStorageClass=Auto  ParallelPVariant=InternalParameters  IdealPVariant=Disabled  IVariant=InternalParameters  DVariant=InternalParameters  IntegratorVariant=Continuous  SatVariant=Disabled  AWVariant=Passthrough  PCopyVariant=Disabled  TRVariant=Disabled  FdbkBlocksVariant=Forward  IdealPFdbkVariant=Disabled  SatFdbkVariant=Disabled  DerivativeFilterVariant=ContFilter  NVariant=InternalParameters  NCopyVariant=Disabled  FilterICVariant=InternalICsFilter  IntegratorICVariant=InternalICs  ExternalResetVariant=Disabled  TRSumVariant=Passthrough  SumFdbkVariant=Disabled  SumVariant=Sum_PID
  Sum1 : Sum  Inputs=++|
  Sum2 : Sum  Inputs=-+|
  T : Outport
  wires:
  z_ref/1 -> Sum2/2  "z_ref"
  Sum2/1 -> PID Controller/1  "z_err"
  z/1 -> Sum2/1  "z"
  PID Controller/1 -> Sum1/2
  Sum1/1 -> T/1  "z_err"
  Constant/1 -> Sum1/1
